simulink model "State_observer"  (R2023b)
settings: Solver=VariableStepAuto  StartTime=0.0  StopTime=30  RelTol=1e-3
values from neighbouring files (symbols this model uses):
  A = double(A)    [consistent.m]    (also in dyn_model_mark.m)
  B = double(B)    [consistent.m]    (also in dyn_model_mark.m)
  C = [1 0 0 0 ... (first row only)    [consistent.m]    (also in dyn_model_mark.m)
  D = [0 ... (first row only)    [consistent.m]    (also in dyn_model_mark.m)
  g0 = 9.81    [consistent.m]    (also in dyn_model_mark.m)
  Ip = (mp*Lp^2)/12    (= 3.3282e-05)    [consistent.m]    (also in dyn_model_mark.m = 8.3205e-06)
  Ir = (mr*Lr^2)/12    (= 5.71979166667e-05)    [consistent.m]    (also in dyn_model_mark.m = 1.42994791667e-05)
  K = place(A,B,P)    [consistent.m]    (also in dyn_model_mark.m)
  L_kf = lqr(A',C',Q_tilde,R_tilde)'    [consistent.m]
  La = 1.16e-3    (= 0.00116)    [consistent.m]    (also in dyn_model_mark.m)
  Lp = 0.129    [consistent.m]    (also in dyn_model_mark.m = 0.0645)
  Lr = 0.085    [consistent.m]    (also in dyn_model_mark.m)
  mp = 0.024    [consistent.m]    (also in dyn_model_mark.m)
  mr = 0.095    [consistent.m]    (also in dyn_model_mark.m)
  phi_dot_init = 0    [consistent.m]
  phi_init = 0    [consistent.m]
  Ra = 8.4    [consistent.m]    (also in dyn_model_mark.m)
  theta_dot_init = 0    [consistent.m]
  theta_init = 0    [consistent.m]
undefined symbols (not defined in the file or in its folder): alfa, beta, dist, Ir_tot, L_pp, Ld, rot_pend
libraries: simulink_extras x8
settings Model: Creator=Mark  LastModifiedBy=Mark

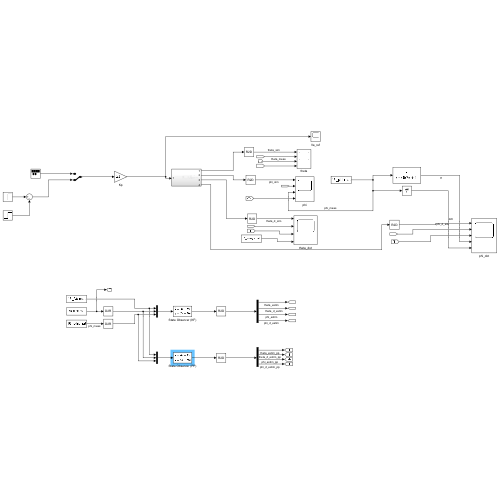
[thumbnail: Simulink's stored preview of the top-level diagram]
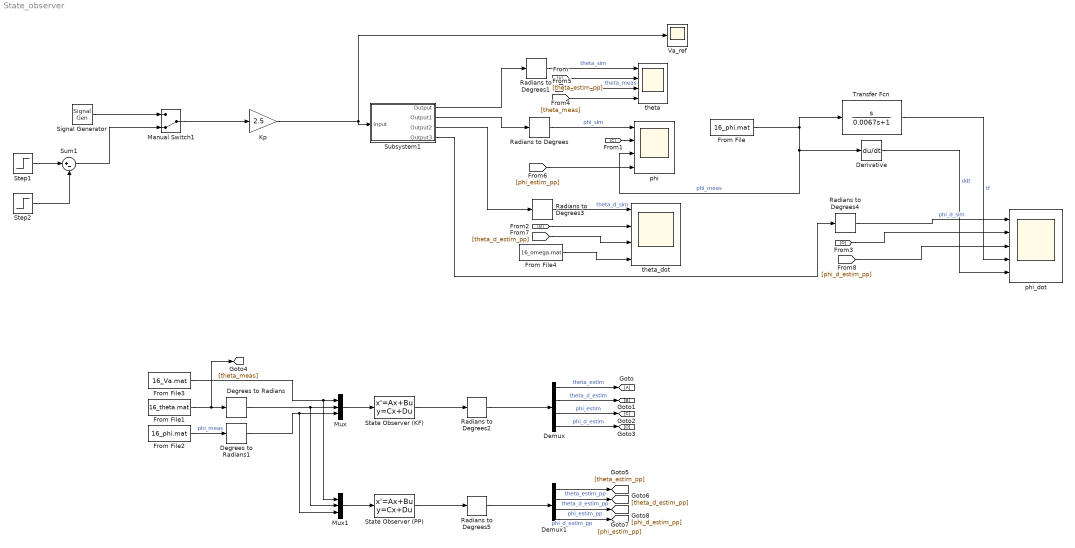
== system State_observer ==
  Degrees to Radians : simulink_extras/Transformations/Degrees to Radians
  Degrees to Radians1 : simulink_extras/Transformations/Degrees to Radians
  Demux : Demux
  Demux1 : Demux
  Derivative : Derivative
  From : From
  From File : FromFile  FileName=16_phi.mat  SampleTime=0
  From File1 : FromFile  FileName=16_theta.mat  SampleTime=0
  From File2 : FromFile  FileName=16_phi.mat  SampleTime=0
  From File3 : FromFile  FileName=16_Va.mat  SampleTime=0
  From File4 : FromFile  FileName=16_omega.mat  SampleTime=0
  Goto : Goto
  Kp : Gain  Gain=2.5
  Manual Switch1 : ManualSwitch  CurrentSetting=0
  Mux : Mux  Inputs=3
  Mux1 : Mux  Inputs=3
  Radians to Degrees{,1..5} (6 alike) : simulink_extras/Transformations/Radians to Degrees
  Signal Generator : SignalGenerator  WaveForm=square  Frequency=0.05
  State Observer (KF) : StateSpace  A=A-L_kf*C  B=[B-L_kf*D L_kf]  C=eye(4)  D=zeros(4,3)  InitialCondition=0  ParameterTunability=Unconstrained
  State Observer (PP) : StateSpace  A=A-L_pp*C  B=[B-L_pp*D L_pp]  C=eye(4)  D=zeros(4,3)  InitialCondition=0
  Step1 : Step  SampleTime=0
  Step2 : Step  Time=1.05  SampleTime=0
  Subsystem1 : Subsystem
  Sum1 : Sum  Inputs=|+-
  Transfer Fcn : TransferFcn  Numerator=[1 0]  Denominator=[0.0067 1]
  Va_ref : Scope
  phi : Scope  NumInputPorts=4
  phi_dot : Scope  NumInputPorts=5
  theta : Scope  NumInputPorts=4
  theta_dot : Scope  NumInputPorts=4
  wires:
  Signal Generator/1 -> Manual Switch1/1
  Manual Switch1/1 -> Kp/1
  Radians to Degrees1/1 -> theta/1  "theta_sim"
  Radians to Degrees/1 -> phi/1  "phi_sim"
  Kp/1 -> Subsystem1/1(Input), Va_ref/1
  Demux/1 -> Goto/1  "theta_estim"
  Demux/2 -> [B]  "theta_d_estim"
  Demux/3 -> [C]  "phi_estim"
  Demux/4 -> [D]  "phi_d_estim"
  From/1 -> theta/2
  [C] -> phi/2
  [B] -> theta_dot/2
  Radians to Degrees2/1 -> Demux/1
  Subsystem1/1(Output) -> Radians to Degrees1/1
  Subsystem1/2(Output1) -> Radians to Degrees/1
  Subsystem1/3(Output2) -> Radians to Degrees3/1
  State Observer (KF)/1 -> Radians to Degrees2/1
  Radians to Degrees3/1 -> theta_dot/1  "theta_d_sim"
  Subsystem1/4(Output3) -> Radians to Degrees4/1
  Radians to Degrees4/1 -> phi_dot/1  "phi_d_sim"
  [D] -> phi_dot/2
  Step1/1 -> Sum1/1
  Sum1/1 -> Manual Switch1/2
  Step2/1 -> Sum1/2
  Mux/1 -> State Observer (KF)/1
  Transfer Fcn/1 -> phi_dot/4  "tf"
  Derivative/1 -> phi_dot/5  "ddt"
  From File/1 -> phi/3, Derivative/1, Transfer Fcn/1  "phi_meas"
  From File1/1 -> [theta_meas], Degrees to Radians/1
  From File2/1 -> Degrees to Radians1/1  "phi_meas"
  From File3/1 -> Mux1/1, Mux/1
  [theta_meas] -> theta/3  "theta_meas"
  Degrees to Radians/1 -> Mux1/2, Mux/2
  Degrees to Radians1/1 -> Mux1/3, Mux/3
  From File4/1 -> theta_dot/4
  Mux1/1 -> State Observer (PP)/1
  State Observer (PP)/1 -> Radians to Degrees5/1
  Radians to Degrees5/1 -> Demux1/1
  Demux1/1 -> [theta_estim_pp]  "theta_estim_pp"
  Demux1/2 -> [theta_d_estim_pp]  "theta_d_estim_pp"
  Demux1/3 -> [phi_estim_pp]  "phi_estim_pp"
  Demux1/4 -> [phi_d_estim_pp]  "phi_d_estim_pp"
  [theta_estim_pp] -> theta/4
  [phi_estim_pp] -> phi/4
  [theta_d_estim_pp] -> theta_dot/3
  [phi_d_estim_pp] -> phi_dot/3

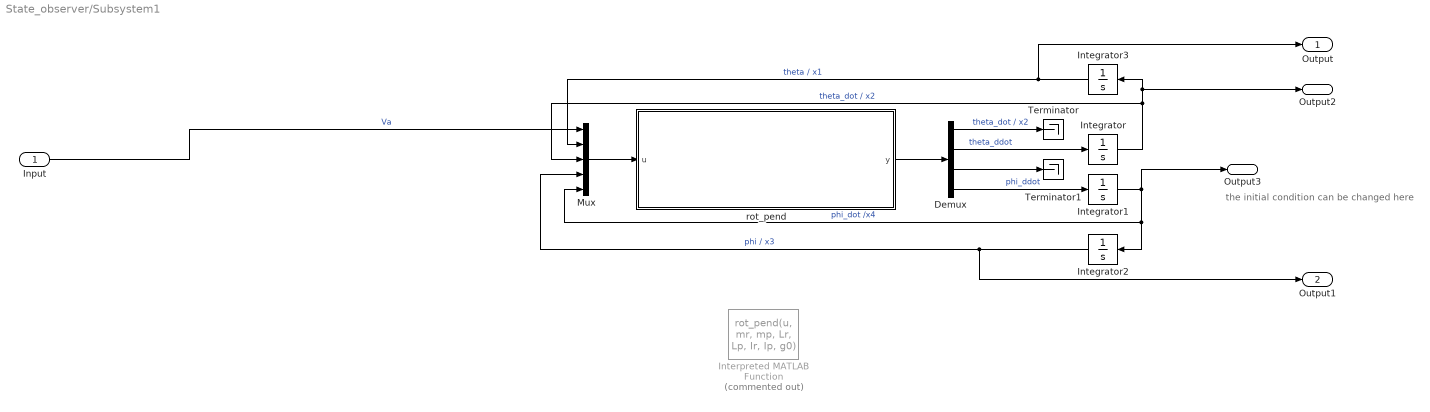
== system State_observer/Subsystem1 ==
  note: the initial condition can be changed here
  Input : Inport
  Demux : Demux
  Integrator : Integrator  InitialCondition=theta_dot_init
  Integrator1 : Integrator  InitialCondition=phi_dot_init
  Integrator2 : Integrator  InitialCondition=phi_init
  Integrator3 : Integrator  InitialCondition=theta_init
  Interpreted MATLAB Function : MATLABFcn  Commented=on  MATLABFcn=rot_pend(u, mr, mp, Lr, Lp, Ir, Ip, g0)  OutputDimensions=4  OutputSignalType=real
  Mux : Mux  Inputs=5
  Terminator : Terminator
  Terminator1 : Terminator
  rot_pend : Subsystem
  Output : Outport
  Output1 : Outport  Port=2
  Output2 : Outport  Port=3
  Output3 : Outport  Port=4
  wires:
  Integrator2/1 -> Output1/1, Mux/4  "phi / x3"
  Integrator/1 -> Integrator3/1, Output2/1, Mux/3  "theta_dot / x2"
  Mux/1 -> rot_pend/1(u)
  rot_pend/1(y) -> Demux/1
  Integrator1/1 -> Output3/1, Mux/5, Integrator2/1  "phi_dot /x4"
  Integrator3/1 -> Mux/2, Output/1  "theta / x1"
  Demux/4 -> Integrator1/1  "phi_ddot"
  Demux/2 -> Integrator/1  "theta_ddot"
  Demux/1 -> Terminator/1  "theta_dot / x2"
  Demux/3 -> Terminator1/1
  Input/1 -> Mux/1  "Va"

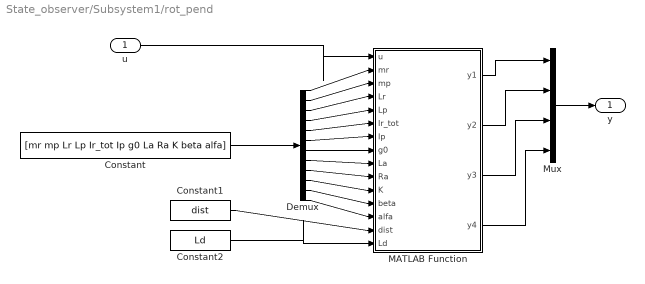
== system State_observer/Subsystem1/rot_pend ==
  u : Inport
  Constant : Constant  Value=[mr mp Lr Lp Ir_tot Ip g0 La Ra K beta alfa]  VectorParams1D=off
  Constant1 : Constant  Value=dist
  Constant2 : Constant  Value=Ld
  Demux : Demux  Outputs=12
  MATLAB Function : MATLAB Function  TreatAsAtomicUnit=on
  Mux : Mux
  y : Outport
  wires:
  Demux/3 -> MATLAB Function/4(Lr)
  Demux/5 -> MATLAB Function/6(Ir_tot)
  Demux/4 -> MATLAB Function/5(Lp)
  Demux/7 -> MATLAB Function/8(g0)
  Demux/2 -> MATLAB Function/3(mp)
  Demux/6 -> MATLAB Function/7(Ip)
  Demux/1 -> MATLAB Function/2(mr)
  u/1 -> MATLAB Function/1(u)
  Constant/1 -> Demux/1
  MATLAB Function/1(y1) -> Mux/1
  MATLAB Function/2(y2) -> Mux/2
  MATLAB Function/3(y3) -> Mux/3
  MATLAB Function/4(y4) -> Mux/4
  Mux/1 -> y/1
  Demux/8 -> MATLAB Function/9(La)
  Demux/9 -> MATLAB Function/10(Ra)
  Demux/10 -> MATLAB Function/11(K)
  Demux/11 -> MATLAB Function/12(beta)
  Constant1/1 -> MATLAB Function/14(dist)
  Constant2/1 -> MATLAB Function/15(Ld)
  Demux/12 -> MATLAB Function/13(alfa)

== matlab function State_observer/Subsystem1/rot_pend/MATLAB Function ==
  data: u input; y1 output; mr input; mp input; Lr input; Lp input; Ir_tot input; Ip input; g0 input; La input; Ra input; y2 output; y3 output; y4 output; K input; beta input; alfa input; dist input; Ld input
function [y1,y2,y3,y4] = rot_pend(u, mr, mp, Lr, Lp, Ir_tot, Ip, g0,La, Ra, K, beta,alfa, dist, Ld)
%UNTITLED Summary of this function goes here
%   Detailed explanation goes here
% u(1) = Va
x1 = u(2) ; % theta
x2 = u(3) ; % theta_dot
x3 = u(4) ; % phi
x4 = u(5) ; % phi_dot

H = [(mp*(Lr^2+((Lp/2)^2*(sin(x3))^2)))+Ir_tot            -mp*Lr*Lp*cos(x3)/2;
                     -mp*Lr*Lp*cos(x3)/2                              (mp*(Lp/2)^2)+Ip] ;

Q = [mp*(Lp/2)^2*sin(x3)*cos(x3)*x4+beta                     (mp*(Lp/2)^2*sin(x3)*cos(x3)*x2)-(mp*Lr*(Lp/2)*sin(x3)*x4);
     -mp*(Lp/2)^2*sin(x3)*cos(x3)*x2                                                   alfa                                   ] ;

g = [           0     ;
     mp*g0*(Lp/2)*sin(x3)] ;
%(K*u(1)/Ra)-(K^2*x2/Ra)
tau = [(K/Ra)*(u(1)-(K*x2)) ;
       0 ] ;

if (x1>=0.1745 | x1<=-0.1745)       % 0.08727rad = 5deg
     kt = 0.03 ;                    % 0.1745rad = 10deg
     kc = 10e-3 ;
else                               % 0.349rad = 20deg
    kt = 0 ;
    kc = 3.5e-3 ;
end
% if (x2>=2.618 | x2<=-2.618)       % 3.49rad/s = 200deg/s
%                                 % 2.618rad/s = 150deg/s
%     kc = 10e-3 ;
% else                               
% 
%     kc = 4.8e-3 ;
% end


Tr_theta = ((kt*x1)+(kc*x2))*Ld ;
q_ddot = H\[tau - Q*[x2 x4]' - g - [Tr_theta 0]' ] ;



y1 = x2 ;
y2 = q_ddot(1) ;
y3 = x4 ;
y4 = q_ddot(2) ;


%Ir+mr*(Lr/2)^2)
